simulink model "testf12"  (R2021b)
settings: Solver=FixedStepAuto  StartTime=91000  StopTime=94788  FixedStep=0.01  RelTol=1e-3
settings Model: Creator=Newsky  LastModifiedBy=Newsky

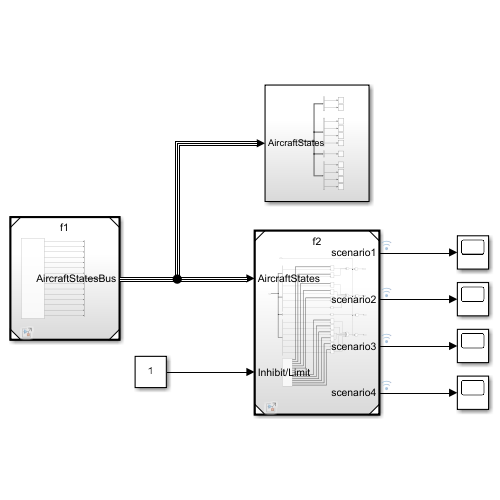
[thumbnail: Simulink's stored preview of the top-level diagram]
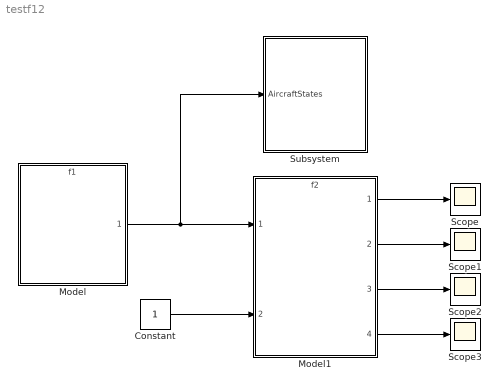
== system testf12 ==
  Constant : Constant  OutDataTypeStr=boolean
  Model : ModelReference  ModelNameDialog=f1.slx  SimulationMode=Normal  ModelReferenceVersion=1.19
  Model1 : ModelReference  ModelNameDialog=f2.slx  SimulationMode=Normal  ModelReferenceVersion=1.16
  Scope{,1..3} (4 alike) : Scope
  Subsystem : Subsystem
  wires:
  Model/1 -> Subsystem/1(AircraftStates), Model1/1
  Model1/1 -> Scope/1
  Model1/2 -> Scope1/1
  Model1/4 -> Scope3/1
  Model1/3 -> Scope2/1
  Constant/1 -> Model1/2

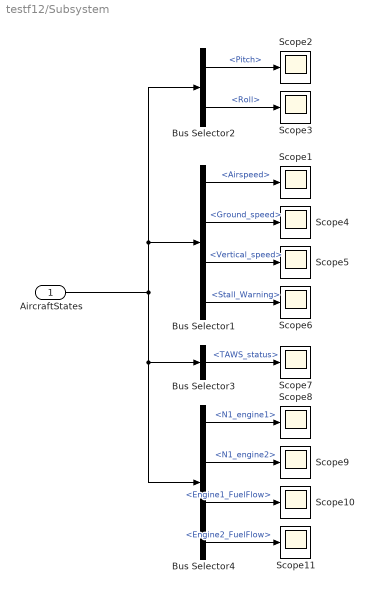
== system testf12/Subsystem ==
  AircraftStates : Inport
  Bus Selector1 : BusSelector  OutputSignals=Airspeed,Ground_speed,Vertical_speed,Stall_Warning
  Bus Selector2 : BusSelector  OutputSignals=Pitch,Roll
  Bus Selector3 : BusSelector  OutputSignals=TAWS_status
  Bus Selector4 : BusSelector  OutputSignals=N1_engine1,N1_engine2,Engine1_FuelFlow,Engine2_FuelFlow
  Scope{1..11} (11 alike) : Scope
  wires:
  Bus Selector2/1 -> Scope2/1  "<Pitch>"
  AircraftStates/1 -> Bus Selector2/1, Bus Selector1/1, Bus Selector4/1, Bus Selector3/1
  Bus Selector2/2 -> Scope3/1  "<Roll>"
  Bus Selector1/1 -> Scope1/1  "<Airspeed>"
  Bus Selector1/2 -> Scope4/1  "<Ground_speed>"
  Bus Selector1/3 -> Scope5/1  "<Vertical_speed>"
  Bus Selector1/4 -> Scope6/1  "<Stall_Warning>"
  Bus Selector3/1 -> Scope7/1  "<TAWS_status>"
  Bus Selector4/4 -> Scope11/1  "<Engine2_FuelFlow>"
  Bus Selector4/3 -> Scope10/1  "<Engine1_FuelFlow>"
  Bus Selector4/2 -> Scope9/1  "<N1_engine2>"
  Bus Selector4/1 -> Scope8/1  "<N1_engine1>"
